simulink model "untitled1"  (R2020b)
settings: Solver=VariableStepAuto  StartTime=0.0  StopTime=10.0  RelTol=1e-3
settings Model: Creator=Yeshwanth  LastModifiedBy=Yeshwanth

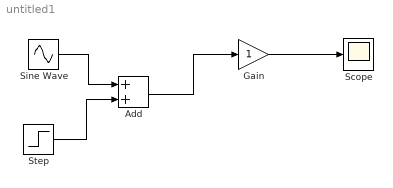
== system untitled1 ==
  Add : Sum
  Gain : Gain
  Scope : Scope
  Sine Wave : Sin  SampleTime=0
  Step : Step  SampleTime=0
  wires:
  Gain/1 -> Scope/1
  Sine Wave/1 -> Add/1
  Step/1 -> Add/2
  Add/1 -> Gain/1
